simulink subsystem "DetailedBatteryModel"  (R2022b)
settings: Solver=VariableStepAuto  StartTime=0.0  StopTime=10.0  RelTol=1e-3
undefined symbols (not defined in the file): PlntBattBalSwtchThresh, PlntBattBleedRes, PlntBattCondArea, PlntBattModNumCellPar
libraries: fl_lib x584, nesl_utility_internal x386, batteryecm_lib x96, simulink x96
(part 6 of 7)

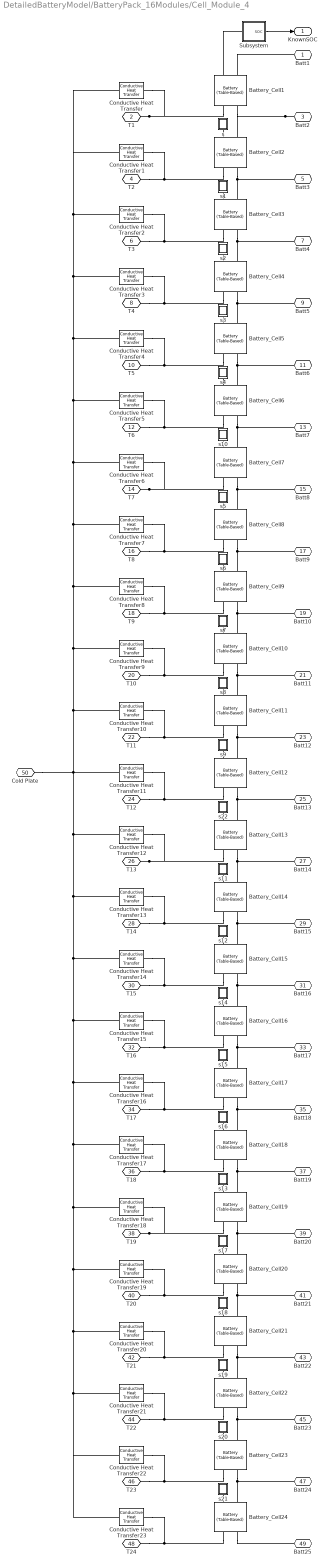
== system DetailedBatteryModel/BatteryPack_16Modules/Cell_Module_4 ==
  Battery_Cell{1..24} (24 alike) : batteryecm_lib/Battery (Table-Based)  Tag={'toolbox/physmod/battery/shared_library/m/batteryecm_lib_parts';'Battery__Table_Based_/Panasonic/NCR18650BD.xml'}  SOC_vec=[0 0.01 0.02 0.03 0.04 0.05 0.06 0.07 0.08 0.09 0.1 0.11 0.12 0.13 0.14 0.15 0.16 0.17 0.18 0.19 0.2 0.21 0.22 0.23 0.24 0.25 0.26 0.27 0.28 0.29 0.3 0.31 0.32 0.33 0.34 0.35 0.36 0.37 0.38 0.39 0.4 0.41 0.42 0.43 0.44 0.45 0.46 0.47 0.48 0.49 0.5 0.51 0.52 0.53 0.54 0.55 0.56 0.57 0.58 0.59 0.6 0.61 0.62 0.63 0.64 0.65 0.66 0.67 0.68 0.69 0.7 0.71 0.72 0.73 0.74 0.75 0.76 0.77 0.78 0.79 0.8 0.81 0.82 0.83 0.84 0.85 0.86 0.87 0.88 0.89 0.9 0.91 0.92 0.93 0.94 0.95 0.96 0.97 0.98 0.99 1]  T_dependence=simscape.enum.tablebattery.temperature_dependence.yes  prm_dir=simscape.enum.tablebattery.prm_dir.noCurrentDirectionality  T_vec=[-10 0 25 40 60] degC  V0_mat=[2.90003 2.90003 2.90003 2.90003 2.90003;2.94341 2.94341 2.94341 2.94341 2.94341;2.98679 2.98679 2.98679 2.98679 2.98679;3.04987 3.04987 3.04987 3.04987 3.04987;3.09433 3.09433 3.09433 3.09433 3.09433;3.12791 3.12791 3.12791 3.12791 3.12791;3.16031 3.16031 3.16031 3.16031 3.16031;3.20369 3.20369 3.20369 3.20369 3.20369;3.23862 3.23862 3.23862 3.23862 3.23862;3.26689 3.26689 3.26689 3.26689 3.26689;3.29115 3.29115 3.29115 3.29115 3.29115;3.31383 3.31383 3.31383 3.31383 3.31383;3.33202 3.33202 3.33202 3.33202 3.33202;3.35112 3.35112 3.35112 3.35112 3.35112;3.36833 3.36833 3.36833 3.36833 3.36833;3.38413 3.38413 3.38413 3.38413 3.38413;3.39973 3.39973 3.39973 3.39973 3.39973;3.41137 3.41137 3.41137 3.41137 3.41137;3.42149 3.42149 3.42149 3.42149 3.42149;3.43136 3.43136 3.43136 3.43136 3.43136;3.44073 3.44073 3.44073 3.44073 3.44073;3.45027 3.45027 3.45027 3.45027 3.45027;3.46068 3.46068 3.46068 3.46068 3.46068;3.47113 3.47113 3.47113 3.47113 3.47113;3.47814 3.47814 3.47814 3.47814 3.47814;3.48494 3.48494 3.48494 3.48494 3.48494;3.49199 3.49199 3.49199 3.49199 3.49199;3.49905 3.49905 3.49905 3.49905 3.49905;3.50562 3.50562 3.50562 3.50562 3.50562;3.51187 3.51187 3.51187 3.51187 3.51187;3.51861 3.51861 3.51861 3.51861 3.51861;3.52535 3.52535 3.52535 3.52535 3.52535;3.53209 3.53209 3.53209 3.53209 3.53209;3.53818 3.53818 3.53818 3.53818 3.53818;3.54353 3.54353 3.54353 3.54353 3.54353;3.54849 3.54849 3.54849 3.54849 3.54849;3.55353 3.55353 3.55353 3.55353 3.55353;3.55855 3.55855 3.55855 3.55855 3.55855;3.56357 3.56357 3.56357 3.56357 3.56357;3.56831 3.56831 3.56831 3.56831 3.56831;3.57308 3.57308 3.57308 3.57308 3.57308;3.57787 3.57787 3.57787 3.57787 3.57787;3.58264 3.58264 3.58264 3.58264 3.58264;3.58755 3.58755 3.58755 3.58755 3.58755;3.5925 3.5925 3.5925 3.5925 3.5925;3.5985 3.5985 3.5985 3.5985 3.5985;3.60496 3.60496 3.60496 3.60496 3.60496;3.61149 3.61149 3.61149 3.61149 3.61149;3.61805 3.61805 3.61805 3.61805 3.61805;3.6246 3.6246 3.6246 3.6246 3.6246;3.63116 3.63116 3.63116 3.63116 3.63116;3.63855 3.63855 3.63855 3.63855 3.63855;3.64609 3.64609 3.64609 3.64609 3.64609;3.65336 3.65336 3.65336 3.65336 3.65336;3.66064 3.66064 3.66064 3.66064 3.66064;3.66791 3.66791 3.66791 3.66791 3.66791;3.67613 3.67613 3.67613 3.67613 3.67613;3.68522 3.68522 3.68522 3.68522 3.68522;3.69443 3.69443 3.69443 3.69443 3.69443;3.70367 3.70367 3.70367 3.70367 3.70367;3.713 3.713 3.713 3.713 3.713;3.72241 3.72241 3.72241 3.72241 3.72241;3.73154 3.73154 3.73154 3.73154 3.73154;3.74037 3.74037 3.74037 3.74037 3.74037;3.7492 3.7492 3.7492 3.7492 3.7492;3.75786 3.75786 3.75786 3.75786 3.75786;3.76617 3.76617 3.76617 3.76617 3.76617;3.77556 3.77556 3.77556 3.77556 3.77556;3.78485 3.78485 3.78485 3.78485 3.78485;3.79413 3.79413 3.79413 3.79413 3.79413;3.8034 3.8034 3.8034 3.8034 3.8034;3.81149 3.81149 3.81149 3.81149 3.81149;3.81977 3.81977 3.81977 3.81977 3.81977;3.82804 3.82804 3.82804 3.82804 3.82804;3.83631 3.83631 3.83631 3.83631 3.83631;3.84472 3.84472 3.84472 3.84472 3.84472;3.85317 3.85317 3.85317 3.85317 3.85317;3.86155 3.86155 3.86155 3.86155 3.86155;3.86993 3.86993 3.86993 3.86993 3.86993;3.87831 3.87831 3.87831 3.87831 3.87831;3.88686 3.88686 3.88686 3.88686 3.88686;3.89534 3.89534 3.89534 3.89534 3.89534;3.90461 3.90461 3.90461 3.90461 3.90461;3.91454 3.91454 3.91454 3.91454 3.91454;3.92565 3.92565 3.92565 3.92565 3.92565;3.93721 3.93721 3.93721 3.93721 3.93721;3.94924 3.94924 3.94924 3.94924 3.94924;3.96155 3.96155 3.96155 3.96155 3.96155;3.97383 3.97383 3.97383 3.97383 3.97383;3.98598 3.98598 3.98598 3.98598 3.98598;3.99856 3.99856 3.99856 3.99856 3.99856;4.01117 4.01117 4.01117 4.01117 4.01117;4.02361 4.02361 4.02361 4.02361 4.02361;4.03609 4.03609 4.03609 4.03609 4.03609;4.04694 4.04694 4.04694 4.04694 4.04694;4.05695 4.05695 4.05695 4.05695 4.05695;4.06641 4.06641 4.06641 4.06641 4.06641;4.07551 4.07551 4.07551 4.07551 4.07551;4.08514 4.08514 4.08514 4.08514 4.08514;4.09447 4.09447 4.09447 4.09447 4.09447;4.10453 4.10453 4.10453 4.10453 4.10453] V  V0_vec=[2.90003 2.94341 2.98679 3.04987 3.09433 3.12791 3.16031 3.20369 3.23862 3.26689 3.29115 3.31383 3.33202 3.35112 3.36833 3.38413 3.39973 3.41137 3.42149 3.43136 3.44073 3.45027 3.46068 3.47113 3.47814 3.48494 3.49199 3.49905 3.50562 3.51187 3.51861 3.52535 3.53209 3.53818 3.54353 3.54849 3.55353 3.55855 3.56357 3.56831 3.57308 3.57787 3.58264 3.58755 3.5925 3.5985 3.60496 3.61149 3.61805 3.6246 3.63116 3.63855 3.64609 3.65336 3.66064 3.66791 3.67613 3.68522 3.69443 3.70367 3.713 3.72241 3.73154 3.74037 3.7492 3.75786 3.76617 3.77556 3.78485 3.79413 3.8034 3.81149 3.81977 3.82804 3.83631 3.84472 3.85317 3.86155 3.86993 3.87831 3.88686 3.89534 3.90461 3.91454 3.92565 3.93721 3.94924 3.96155 3.97383 3.98598 3.99856 4.01117 4.02361 4.03609 4.04694 4.05695 4.06641 4.07551 4.08514 4.09447 4.10453] V  V_range=[2.25 Inf] V  R0_mat=[0.54124 0.47218 0.1741 0.16472 0.13072;0.60048 0.51942 0.15823 0.09801 0.03241;0.57827 0.49613 0.14313 0.06257 0.00499;0.55606 0.47283 0.13285 0.0492 0.00058;0.53384 0.44953 0.12044 0.03857 0.00058;0.51163 0.42624 0.10641 0.0337 0.00058;0.48942 0.40294 0.09605 0.03258 0.00058;0.46721 0.37965 0.09162 0.03508 0.0103;0.44499 0.35635 0.08758 0.0376 0.01722;0.42278 0.33305 0.08349 0.04115 0.02235;0.40057 0.30976 0.08021 0.04338 0.0273;0.37836 0.28646 0.07738 0.04509 0.03173;0.35615 0.26317 0.07487 0.04551 0.03469;0.33393 0.24021 0.07338 0.04781 0.03783;0.31172 0.21801 0.07189 0.04948 0.04012;0.28951 0.203 0.07117 0.05069 0.04195;0.26873 0.19013 0.0704 0.05182 0.04371;0.24946 0.17834 0.06898 0.05166 0.04417;0.23189 0.16793 0.06755 0.05143 0.04397;0.21926 0.15878 0.06631 0.0513 0.04362;0.2084 0.15119 0.06509 0.05101 0.04311;0.19882 0.14534 0.06388 0.05077 0.04265;0.19282 0.14029 0.06326 0.05091 0.04272;0.18782 0.13679 0.06281 0.05124 0.04325;0.18252 0.13215 0.06182 0.05043 0.04264;0.17725 0.12766 0.06095 0.04955 0.04196;0.173 0.125 0.06025 0.04876 0.04137;0.16875 0.12234 0.05955 0.04802 0.04078;0.16459 0.11952 0.05877 0.04782 0.04033;0.16124 0.11704 0.05807 0.04752 0.03993;0.15805 0.11494 0.05761 0.04737 0.03969;0.15486 0.11285 0.05714 0.04723 0.03945;0.15212 0.11075 0.05668 0.04709 0.03921;0.15022 0.10906 0.05611 0.04673 0.03878;0.14807 0.10773 0.05546 0.04612 0.03867;0.14579 0.10628 0.0549 0.04546 0.03843;0.14353 0.10484 0.05439 0.04485 0.03821;0.14127 0.10351 0.05388 0.04423 0.03799;0.13957 0.10228 0.05337 0.04361 0.03777;0.13785 0.10097 0.0528 0.0429 0.03746;0.13614 0.09966 0.05223 0.0422 0.0367;0.13443 0.09836 0.05165 0.04151 0.03572;0.13272 0.09711 0.05106 0.04111 0.03474;0.13096 0.09591 0.05046 0.04079 0.03381;0.12918 0.09471 0.04986 0.04049 0.03288;0.12775 0.09387 0.04945 0.04053 0.03231;0.12648 0.09317 0.04913 0.04073 0.03189;0.12522 0.09249 0.04883 0.04095 0.03151;0.12398 0.09181 0.04854 0.04066 0.03136;0.12296 0.09112 0.04826 0.04006 0.03121;0.12207 0.09044 0.04797 0.03947 0.03106;0.12147 0.09003 0.04782 0.03916 0.03119;0.12091 0.08967 0.04765 0.03889 0.03136;0.12027 0.08886 0.0473 0.03854 0.03145;0.11955 0.08797 0.04695 0.03818 0.03154;0.11836 0.08708 0.04661 0.03764 0.03136;0.11749 0.08651 0.04638 0.03733 0.03126;0.1169 0.08628 0.0463 0.03731 0.03144;0.11636 0.0866 0.04625 0.03733 0.03167;0.11679 0.08693 0.04621 0.03736 0.0319;0.11639 0.08729 0.04624 0.03741 0.03216;0.11602 0.08748 0.04628 0.0375 0.03245;0.11556 0.08747 0.04628 0.03749 0.03262;0.115 0.08737 0.04623 0.03738 0.03268;0.11444 0.08726 0.04617 0.03728 0.03275;0.11413 0.08683 0.04599 0.03714 0.03276;0.11369 0.08629 0.04573 0.03712 0.03265;0.11362 0.0861 0.0457 0.03746 0.03289;0.11351 0.08597 0.04568 0.03777 0.03289;0.1134 0.08596 0.04565 0.03807 0.03285;0.11329 0.08593 0.04563 0.03837 0.0328;0.11297 0.08552 0.04535 0.03804 0.03236;0.1131 0.0855 0.0451 0.03769 0.03198;0.11323 0.08564 0.04486 0.03733 0.0316;0.11336 0.08578 0.04461 0.03698 0.03122;0.11354 0.08596 0.04446 0.03667 0.03091;0.11376 0.08614 0.04435 0.03629 0.0306;0.11421 0.08628 0.04423 0.03577 0.03027;0.11467 0.08641 0.04411 0.03525 0.02995;0.11513 0.08655 0.044 0.03473 0.02961;0.11565 0.08679 0.04372 0.03426 0.02933;0.11614 0.08704 0.04339 0.03378 0.02903;0.11689 0.08756 0.04323 0.03353 0.02899;0.11825 0.08829 0.0432 0.03328 0.02916;0.12033 0.08941 0.04344 0.03342 0.02973;0.12256 0.09067 0.04374 0.03371 0.0301;0.12495 0.09191 0.0441 0.03415 0.02981;0.12743 0.09323 0.04452 0.03468 0.0296;0.13108 0.09454 0.04494 0.03488 0.02939;0.13509 0.09581 0.0454 0.03488 0.02914;0.13924 0.09835 0.04594 0.03502 0.02907;0.14357 0.1012 0.0463 0.03517 0.02937;0.14857 0.10399 0.04649 0.03528 0.02963;0.15358 0.10679 0.04668 0.03541 0.02989;0.15894 0.10894 0.04629 0.035 0.02961;0.16451 0.11073 0.04541 0.03434 0.02892;0.17255 0.11235 0.04438 0.03375 0.02804;0.17994 0.11383 0.04326 0.03305 0.02704;0.18615 0.11422 0.04154 0.03252 0.02601;0.19123 0.11362 0.03869 0.03189 0.02484;0.17773 0.09538 0.03326 0.0315 0.0239]./PlntBattModNumCellPar Ohm  R0_vec=[0.1741 0.15823 0.14313 0.13285 0.12044 0.10641 0.09605 0.09162 0.08758 0.08349 0.08021 0.07738 0.07487 0.07338 0.07189 0.07117 0.0704 0.06898 0.06755 0.06631 0.06509 0.06388 0.06326 0.06281 0.06182 0.06095 0.06025 0.05955 0.05877 0.05807 0.05761 0.05714 0.05668 0.05611 0.05546 0.0549 0.05439 0.05388 0.05337 0.0528 0.05223 0.05165 0.05106 0.05046 0.04986 0.04945 0.04913 0.04883 0.04854 0.04826 0.04797 0.04782 0.04765 0.0473 0.04695 0.04661 0.04638 0.0463 0.04625 0.04621 0.04624 0.04628 0.04628 0.04623 0.04617 0.04599 0.04573 0.0457 0.04568 0.04565 0.04563 0.04535 0.0451 0.04486 0.04461 0.04446 0.04435 0.04423 0.04411 0.044 0.04372 0.04339 0.04323 0.0432 0.04344 0.04374 0.0441 0.04452 0.04494 0.0454 0.04594 0.0463 0.04649 0.04668 0.04629 0.04541 0.04438 0.04326 0.04154 0.03869 0.03326] Ohm  R0_dis_mat=[.0117, .0085, .009; .011, .0085, .009; .0114, .0087, .0092; .0107, .0082, .0088; .0107, .0083, .0091; .0113, .0085, .0089; .0116, .0085, .0089]./PlntBattModNumCellPar % Parameter not set Ohm  R0_dis_vec=[.0085, .0085, .0087, .0082, .0083, .0085, .0085] % Parameter not set Ohm  R0_ch_mat=[.0117, .0085, .009; .011, .0085, .009; .0114, .0087, .0092; .0107, .0082, .0088; .0107, .0083, .0091; .0113, .0085, .0089; .0116, .0085, .0089]./PlntBattModNumCellPar % Parameter not set Ohm  R0_ch_vec=[.0085, .0085, .0087, .0082, .0083, .0085, .0085] % Parameter not set Ohm  AH=3.153*PlntBattModNumCellPar hr*A  prm_leak=simscape.enum.tablebattery.prm_leak.disabled  Rleak_vec=[8000, 7000, 6000] % Parameter not set Ohm  Rleak=7e3 % Parameter not set Ohm  extrapolation_option=simscape.enum.extrapolation.nearest  SOC_port=simscape.enum.tablebattery.enable.yes  prm_dyn=simscape.enum.tablebattery.prm_dyn.off  R1_mat=[.0109, .0029, .0013; .0069, .0024, .0012; .0047, .0026, .0013; .0034, .0016, .001; .0033, .0023, .0014; .0033, .0018, .0011; .0028, .0017, .0011] % Parameter not set Ohm  R1_vec=[.0029, .0024, .0026, .0016, .0023, .0018, .0017] % Parameter not set Ohm  tau1_mat=[20, 36, 39; 31, 45, 39; 109, 105, 61; 36, 29, 26; 59, 77, 67; 40, 33, 29; 25, 39, 33] % Parameter not set s  tau1_vec=[36, 45, 105, 29, 77, 33, 39] % Parameter not set s  R2_mat=[.0109, .0029, .0013; .0069, .0024, .0012; .0047, .0026, .0013; .0034, .0016, .001; .0033, .0023, .0014; .0033, .0018, .0011; .0028, .0017, .0011] % Parameter not set Ohm  R2_vec=[.0029, .0024, .0026, .0016, .0023, .0018, .0017] % Parameter not set Ohm  tau2_mat=[20, 36, 39; 31, 45, 39; 109, 105, 61; 36, 29, 26; 59, 77, 67; 40, 33, 29; 25, 39, 33] % Parameter not set s  tau2_vec=[36, 45, 105, 29, 77, 33, 39] % Parameter not set s  R3_mat=[.0109, .0029, .0013; .0069, .0024, .0012; .0047, .0026, .0013; .0034, .0016, .001; .0033, .0023, .0014; .0033, .0018, .0011; .0028, .0017, .0011] % Parameter not set Ohm  R3_vec=[.0029, .0024, .0026, .0016, .0023, .0018, .0017] % Parameter not set Ohm  tau3_mat=[20, 36, 39; 31, 45, 39; 109, 105, 61; 36, 29, 26; 59, 77, 67; 40, 33, 29; 25, 39, 33] % Parameter not set s  tau3_vec=[36, 45, 105, 29, 77, 33, 39] % Parameter not set s  R4_mat=[.0109, .0029, .0013; .0069, .0024, .0012; .0047, .0026, .0013; .0034, .0016, .001; .0033, .0023, .0014; .0033, .0018, .0011; .0028, .0017, .0011] % Parameter not set Ohm  R4_vec=[.0029, .0024, .0026, .0016, .0023, .0018, .0017] % Parameter not set Ohm  tau4_mat=[20, 36, 39; 31, 45, 39; 109, 105, 61; 36, 29, 26; 59, 77, 67; 40, 33, 29; 25, 39, 33] % Parameter not set s  tau4_vec=[36, 45, 105, 29, 77, 33, 39] % Parameter not set s  R5_mat=[.0109, .0029, .0013; .0069, .0024, .0012; .0047, .0026, .0013; .0034, .0016, .001; .0033, .0023, .0014; .0033, .0018, .0011; .0028, .0017, .0011] % Parameter not set Ohm  R5_vec=[.0029, .0024, .0026, .0016, .0023, .0018, .0017] % Parameter not set Ohm  tau5_mat=[20, 36, 39; 31, 45, 39; 109, 105, 61; 36, 29, 26; 59, 77, 67; 40, 33, 29; 25, 39, 33] % Parameter not set s  tau5_vec=[36, 45, 105, 29, 77, 33, 39] % Parameter not set s  prm_fade=simscape.enum.tablebattery.prm_fade.disabled  N0=100 % Parameter not set  dV0=0 % Parameter not set  dR0=0 % Parameter not set  dAH=0 % Parameter not set  dRleak=0 % Parameter not set  dR1=0 % Parameter not set  dR2=0 % Parameter not set  dR3=0 % Parameter not set  dR4=0 % Parameter not set  dR5=0 % Parameter not set  N0vec=[1 5 9 13 17 21 25 29 33 37 41 45 49 53 57 61 65 69 73 77 81 85 89 93 97 101 105 109 113 117 121 125 129 133 137 141 145 149 153 157 161 165 169 173 177 181 185 189 193 197 201 205 209 213 217 221 225 229 233 237 241 245 249 253 257 261 265 269 273 277 281 285 289 293 297 301 305 309 313 317]  Tfadevec=[298.15, 323.15] % Parameter not set K  dV0vec=[0 -0.2107 -0.4072 -0.4916 -0.5781 -0.6646 -0.7487 -0.8154 -0.8801 -0.9454 -1.0127 -1.08 -1.1384 -1.1799 -1.2225 -1.2652 -1.3079 -1.3505 -1.3932 -1.4386 -1.4849 -1.5273 -1.567 -1.6067 -1.6464 -1.6889 -1.7346 -1.7803 -1.826 -1.8717 -1.9175 -1.9634 -2.0091 -2.0549 -2.1006 -2.1463 -2.1921 -2.2378 -2.2801 -2.3167 -2.3534 -2.39 -2.4267 -2.4633 -2.4999 -2.5366 -2.5732 -2.6098 -2.6449 -2.6793 -2.7137 -2.7482 -2.7826 -2.817 -2.8515 -2.8859 -2.9192 -2.9512 -2.9793 -3.0074 -3.0355 -3.0636 -3.0917 -3.1198 -3.1479 -3.1758 -3.2018 -3.2279 -3.254 -3.2801 -3.3062 -3.3323 -3.3605 -3.3912 -3.4219 -3.4526 -3.4833 -3.5141 -3.5449 -3.5756]  dR0vec=[0 0 0 0 0 0 0 0 0 0 0 0 0 0 0 0 0 0 0 0 0 0 0 0 0 0 0 0 0 0 0 0 0 0 0 0 0 0 0 0 0 0 0 0 0 0 0 0 0 0 0 0 0 0 0 0 0 0 0 0 0 0 0 0 0 0 0 0 0 0 0 0 0 0 0 0 0 0 0 0] % Parameter assumed  dAHvec=[0 -0.86 -1.713 -2.082 -2.451 -2.819 -3.188 -3.489 -3.781 -4.073 -4.365 -4.657 -4.91 -5.085 -5.26 -5.435 -5.61 -5.785 -5.96 -6.135 -6.31 -6.47 -6.62 -6.771 -6.921 -7.071 -7.221 -7.371 -7.522 -7.672 -7.822 -7.973 -8.124 -8.275 -8.426 -8.577 -8.728 -8.879 -9.018 -9.137 -9.256 -9.376 -9.495 -9.614 -9.734 -9.853 -9.972 -10.091 -10.206 -10.318 -10.431 -10.543 -10.655 -10.768 -10.88 -10.992 -11.105 -11.213 -11.308 -11.403 -11.498 -11.593 -11.687 -11.782 -11.877 -11.972 -12.059 -12.146 -12.233 -12.321 -12.408 -12.495 -12.589 -12.692 -12.794 -12.897 -12.999 -13.102 -13.205 -13.307]  dRleakvec=[0, 0, 0] % Parameter not set  dR1vec=[0, 0, 0] % Parameter not set  dR2vec=[0, 0, 0] % Parameter not set  dR3vec=[0, 0, 0] % Parameter not set  dR4vec=[0, 0, 0] % Parameter not set  dR5vec=[0, 0, 0] % Parameter not set  dV0mat=[0, 0; 0, 0; 0, 0] % Parameter not set  dR0mat=[0, 0; 0, 0; 0, 0] % Parameter not set  dAHmat=[0, 0; 0, 0; 0, 0] % Parameter not set  dRleakmat=[0, 0; 0, 0; 0, 0] % Parameter not set  dR1mat=[0, 0; 0, 0; 0, 0] % Parameter not set  dR2mat=[0, 0; 0, 0; 0, 0] % Parameter not set  dR3mat=[0, 0; 0, 0; 0, 0] % Parameter not set  dR4mat=[0, 0; 0, 0; 0, 0] % Parameter not set  dR5mat=[0, 0; 0, 0; 0, 0] % Parameter not set  prm_age_modeling=simscape.enum.tablebattery.prm_age_modeling.equation  storage_dt_age_vec=[0] % Parameter not set d  storage_T_age_vec=[273] % Parameter not set K  prm_age_OCV=simscape.enum.tablebattery.prm_age_OCV.OCV  OCV_age=0.9 % Parameter not set  SOC_age=0.6 % Parameter not set  prm_age_resistance=simscape.enum.tablebattery.prm_age.disabled  OCV_scaling_age_resistance=2.2134e6 % Parameter not set  OCV_offset_age_resistance=1.632e6 % Parameter not set  temp_exp_age_resistance=0.515833569 % Parameter not set V  t_exp_age_resistance=0.75 % Parameter not set  T_age_vec_resistance=[273.15, 298.15, 323.15] % Parameter not set K  dt_age_vec_resistance=[90, 180, 270, 360] % Parameter not set d  dR0_age_vec=[0, 0, 0] % Parameter not set  t_meas_dR0_age=100 % Parameter not set d  dR0_age_mat=[0, 0, 0; 0, 0, 0; 0, 0, 0; 0, 0, 0] % Parameter not set  prm_age_capacity=simscape.enum.tablebattery.prm_age.disabled  OCV_scaling_age_capacity=1.5097e07 % Parameter not set  OCV_offset_age_capacity=8.3625e06 % Parameter not set  temp_exp_age_capacity=0.6011 % Parameter not set V  t_exp_age_capacity=0.75 % Parameter not set  T_age_vec_capacity=[273.15, 298.15, 323.15] % Parameter not set K  dt_age_vec_capacity=[90, 180, 270, 360] % Parameter not set d  dAH_age_vec=[0, 0, 0] % Parameter not set  t_meas_dAH_age=100 % Parameter not set d  dAH_age_mat=[0, 0, 0; 0, 0, 0; 0, 0, 0; 0, 0, 0] % Parameter not set  thermal_port=simscape.enum.thermaleffects.model  temperature=298.15 % Parameter not set K  thermal_mass=44.55*PlntBattModNumCellPar % Parameter assumed J/K  i_specify=off  i_priority=None  i=0 A  i_nominal_specify=off  i_nominal_unit=A  i_nominal_value=1  v_specify=off  v_priority=None  v=0 V  v_nominal_specify=off  v_nominal_unit=V  v_nominal_value=1  stateOfCharge_specify=on  stateOfCharge_priority=High  stateOfCharge=PlntBattSocInit  stateOfCharge_nominal_specify=off  stateOfCharge_nominal_unit=1  stateOfCharge_nominal_value=1  num_cycles_specify=off  num_cycles_priority=High  num_cycles=0  num_cycles_nominal_specify=off  num_cycles_nominal_unit=1  num_cycles_nominal_value=1  cell_temperature_specify=on  cell_temperature_priority=High  cell_temperature=PlntBattTempInitDegC degC  cell_temperature_nominal_specify=off  cell_temperature_nominal_unit=K  cell_temperature_nominal_value=1
      settings: AttributesFormatString=Panasonic:NCR18650BD
  Conductive Heat Transfer{,1..23} (24 alike) : fl_lib/Thermal/Thermal Elements/Conductive Heat Transfer  thermal_type=foundation.enum.ConstantVariableTabulated.Constant  wall_geometry=foundation.enum.ConductionWallGeometry.Planar  area=PlntBattCondArea*PlntBattModNumCellPar m^2  thickness=PlntBattCondThick m  d_in=0.05 m  d_out=0.1 m  L=1 m  th_cond_min=10 W/(K*m)  th_cond=PlntBattThermCond W/(m*K)  th_cond_TLU=[413, 401, 392, 383, 371, 357, 342] W/(K*m)  temp_TLU=[200, 273, 400, 600, 800, 1000, 1200] K  T_specify=off  T_priority=None  T=0 K  T_nominal_specify=off  T_nominal_unit=K  T_nominal_value=1  Q_specify=off  Q_priority=None  Q=0 W  Q_nominal_specify=off  Q_nominal_unit=W  Q_nominal_value=1
  Subsystem : Subsystem
  s : Subsystem
  s1 : Subsystem
  s10 : Subsystem
  s11 : Subsystem
  s12 : Subsystem
  s13 : Subsystem
  s14 : Subsystem
  s15 : Subsystem
  s16 : Subsystem
  s17 : Subsystem
  s18 : Subsystem
  s19 : Subsystem
  s2 : Subsystem
  s20 : Subsystem
  s21 : Subsystem
  s22 : Subsystem
  s3 : Subsystem
  s4 : Subsystem
  s5 : Subsystem
  s6 : Subsystem
  s7 : Subsystem
  s8 : Subsystem
  s9 : Subsystem
  Batt1 : PMIOPort  Side=Right
  T1 : PMIOPort  Port=2  Side=Right
  Batt2 : PMIOPort  Port=3  Side=Right
  T2 : PMIOPort  Port=4  Side=Right
  Batt3 : PMIOPort  Port=5  Side=Right
  T3 : PMIOPort  Port=6  Side=Right
  Batt4 : PMIOPort  Port=7  Side=Right
  T4 : PMIOPort  Port=8  Side=Right
  Batt5 : PMIOPort  Port=9  Side=Right
  T5 : PMIOPort  Port=10  Side=Right
  Batt6 : PMIOPort  Port=11  Side=Right
  T6 : PMIOPort  Port=12  Side=Right
  Batt7 : PMIOPort  Port=13  Side=Right
  T7 : PMIOPort  Port=14  Side=Right
  Batt8 : PMIOPort  Port=15  Side=Right
  T8 : PMIOPort  Port=16  Side=Right
  Batt9 : PMIOPort  Port=17  Side=Right
  T9 : PMIOPort  Port=18  Side=Right
  Batt10 : PMIOPort  Port=19  Side=Right
  T10 : PMIOPort  Port=20  Side=Right
  Batt11 : PMIOPort  Port=21  Side=Right
  T11 : PMIOPort  Port=22  Side=Right
  Batt12 : PMIOPort  Port=23  Side=Right
  T12 : PMIOPort  Port=24  Side=Right
  Batt13 : PMIOPort  Port=25  Side=Right
  T13 : PMIOPort  Port=26  Side=Right
  Batt14 : PMIOPort  Port=27  Side=Right
  T14 : PMIOPort  Port=28  Side=Right
  Batt15 : PMIOPort  Port=29  Side=Right
  T15 : PMIOPort  Port=30  Side=Right
  Batt16 : PMIOPort  Port=31  Side=Right
  T16 : PMIOPort  Port=32  Side=Right
  Batt17 : PMIOPort  Port=33  Side=Right
  T17 : PMIOPort  Port=34  Side=Right
  Batt18 : PMIOPort  Port=35  Side=Right
  T18 : PMIOPort  Port=36  Side=Right
  Batt19 : PMIOPort  Port=37  Side=Right
  T19 : PMIOPort  Port=38  Side=Right
  Batt20 : PMIOPort  Port=39  Side=Right
  T20 : PMIOPort  Port=40  Side=Right
  Batt21 : PMIOPort  Port=41  Side=Right
  T21 : PMIOPort  Port=42  Side=Right
  Batt22 : PMIOPort  Port=43  Side=Right
  T22 : PMIOPort  Port=44  Side=Right
  Batt23 : PMIOPort  Port=45  Side=Right
  T23 : PMIOPort  Port=46  Side=Right
  Batt24 : PMIOPort  Port=47  Side=Right
  T24 : PMIOPort  Port=48  Side=Right
  Batt25 : PMIOPort  Port=49  Side=Right
  Cold Plate : PMIOPort  Port=50  Side=Left
  KnownSOC : Outport
  wires:
  Subsystem/1(soc) -> KnownSOC/1
  connections:
  T4/RConn1 -- Conductive Heat Transfer3/LConn1 -- Battery_Cell4/RConn2
  T2/RConn1 -- Conductive Heat Transfer1/LConn1 -- Battery_Cell2/RConn2
  T3/RConn1 -- Conductive Heat Transfer2/LConn1 -- Battery_Cell3/RConn2
  Battery_Cell6/LConn2 -- s4/LConn1
  Battery_Cell5/LConn2 -- s3/LConn1
  Battery_Cell4/LConn2 -- s2/LConn1
  Battery_Cell3/LConn2 -- s1/LConn1
  Battery_Cell2/LConn2 -- s/LConn1
  Battery_Cell1/LConn2 -- Subsystem/LConn1
  Battery_Cell2/RConn1 -- Batt3/RConn1 -- Battery_Cell3/LConn1
  Battery_Cell1/LConn1 -- Batt1/RConn1
  Battery_Cell6/RConn1 -- Batt7/RConn1 -- Battery_Cell7/LConn1
  Conductive Heat Transfer12/RConn1 -- Conductive Heat Transfer13/RConn1 -- Conductive Heat Transfer14/RConn1 -- Conductive Heat Transfer15/RConn1 -- Conductive Heat Transfer16/RConn1 -- Conductive Heat Transfer17/RConn1 -- Conductive Heat Transfer18/RConn1 -- Conductive Heat Transfer19/RConn1 -- Conductive Heat Transfer20/RConn1 -- Conductive Heat Transfer21/RConn1 -- Conductive Heat Transfer23/RConn1 -- Conductive Heat Transfer22/RConn1 -- Conductive Heat Transfer11/RConn1 -- Conductive Heat Transfer10/RConn1 -- Conductive Heat Transfer9/RConn1 -- Conductive Heat Transfer8/RConn1 -- Conductive Heat Transfer7/RConn1 -- Conductive Heat Transfer6/RConn1 -- Conductive Heat Transfer5/RConn1 -- Conductive Heat Transfer4/RConn1 -- Conductive Heat Transfer3/RConn1 -- Conductive Heat Transfer2/RConn1 -- Conductive Heat Transfer1/RConn1 -- Conductive Heat Transfer/RConn1 -- Cold Plate/RConn1
  T6/RConn1 -- Conductive Heat Transfer5/LConn1 -- Battery_Cell6/RConn2
  Batt2/RConn1 -- Battery_Cell1/RConn1 -- Battery_Cell2/LConn1
  T5/RConn1 -- Conductive Heat Transfer4/LConn1 -- Battery_Cell5/RConn2
  T1/RConn1 -- Battery_Cell1/RConn2 -- Conductive Heat Transfer/LConn1
  Battery_Cell3/RConn1 -- Batt4/RConn1 -- Battery_Cell4/LConn1
  Battery_Cell5/RConn1 -- Batt6/RConn1 -- Battery_Cell6/LConn1
  Battery_Cell4/RConn1 -- Batt5/RConn1 -- Battery_Cell5/LConn1
  T7/RConn1 -- Conductive Heat Transfer6/LConn1 -- Battery_Cell7/RConn2
  Battery_Cell7/RConn1 -- Batt8/RConn1 -- Battery_Cell8/LConn1
  T12/RConn1 -- Conductive Heat Transfer11/LConn1 -- Battery_Cell12/RConn2
  Battery_Cell11/RConn1 -- Batt12/RConn1 -- Battery_Cell12/LConn1
  Battery_Cell8/RConn1 -- Batt9/RConn1 -- Battery_Cell9/LConn1
  T10/RConn1 -- Conductive Heat Transfer9/LConn1 -- Battery_Cell10/RConn2
  Battery_Cell10/RConn1 -- Batt11/RConn1 -- Battery_Cell11/LConn1
  Battery_Cell9/RConn1 -- Batt10/RConn1 -- Battery_Cell10/LConn1
  T11/RConn1 -- Conductive Heat Transfer10/LConn1 -- Battery_Cell11/RConn2
  T8/RConn1 -- Conductive Heat Transfer7/LConn1 -- Battery_Cell8/RConn2
  T9/RConn1 -- Conductive Heat Transfer8/LConn1 -- Battery_Cell9/RConn2
  Battery_Cell11/LConn2 -- s8/LConn1
  Battery_Cell12/RConn1 -- Batt13/RConn1 -- Battery_Cell13/LConn1
  Battery_Cell10/LConn2 -- s7/LConn1
  Battery_Cell12/LConn2 -- s9/LConn1
  Battery_Cell8/LConn2 -- s5/LConn1
  Battery_Cell9/LConn2 -- s6/LConn1
  Battery_Cell7/LConn2 -- s10/LConn1
  Battery_Cell19/RConn1 -- Batt20/RConn1 -- Battery_Cell20/LConn1
  Battery_Cell13/RConn1 -- Batt14/RConn1 -- Battery_Cell14/LConn1
  T18/RConn1 -- Conductive Heat Transfer17/LConn1 -- Battery_Cell18/RConn2
  Battery_Cell20/RConn1 -- Batt21/RConn1 -- Battery_Cell21/LConn1
  T16/RConn1 -- Conductive Heat Transfer15/LConn1 -- Battery_Cell16/RConn2
  Battery_Cell15/RConn1 -- Batt16/RConn1 -- Battery_Cell16/LConn1
  Battery_Cell23/RConn1 -- Batt24/RConn1 -- Battery_Cell24/LConn1
  T14/RConn1 -- Conductive Heat Transfer13/LConn1 -- Battery_Cell14/RConn2
  T21/RConn1 -- Conductive Heat Transfer20/LConn1 -- Battery_Cell21/RConn2
  T20/RConn1 -- Conductive Heat Transfer19/LConn1 -- Battery_Cell20/RConn2
  Battery_Cell16/RConn1 -- Batt17/RConn1 -- Battery_Cell17/LConn1
  Battery_Cell22/RConn1 -- Batt23/RConn1 -- Battery_Cell23/LConn1
  Battery_Cell17/RConn1 -- Batt18/RConn1 -- Battery_Cell18/LConn1
  T22/RConn1 -- Conductive Heat Transfer21/LConn1 -- Battery_Cell22/RConn2
  T24/RConn1 -- Conductive Heat Transfer23/LConn1 -- Battery_Cell24/RConn2
  T15/RConn1 -- Conductive Heat Transfer14/LConn1 -- Battery_Cell15/RConn2
  T13/RConn1 -- Conductive Heat Transfer12/LConn1 -- Battery_Cell13/RConn2
  T17/RConn1 -- Conductive Heat Transfer16/LConn1 -- Battery_Cell17/RConn2
  Battery_Cell21/RConn1 -- Batt22/RConn1 -- Battery_Cell22/LConn1
  Battery_Cell18/RConn1 -- Batt19/RConn1 -- Battery_Cell19/LConn1
  T19/RConn1 -- Conductive Heat Transfer18/LConn1 -- Battery_Cell19/RConn2
  T23/RConn1 -- Conductive Heat Transfer22/LConn1 -- Battery_Cell23/RConn2
  Battery_Cell14/RConn1 -- Batt15/RConn1 -- Battery_Cell15/LConn1
  Battery_Cell22/LConn2 -- s19/LConn1
  Battery_Cell17/LConn2 -- s15/LConn1
  Battery_Cell16/LConn2 -- s14/LConn1
  Battery_Cell24/LConn2 -- s21/LConn1
  Battery_Cell20/LConn2 -- s17/LConn1
  Battery_Cell18/LConn2 -- s16/LConn1
  Battery_Cell23/LConn2 -- s20/LConn1
  Battery_Cell14/LConn2 -- s11/LConn1
  Battery_Cell19/LConn2 -- s13/LConn1
  Battery_Cell15/LConn2 -- s12/LConn1
  Battery_Cell24/RConn1 -- Batt25/RConn1
  Battery_Cell21/LConn2 -- s18/LConn1
  Battery_Cell13/LConn2 -- s22/LConn1

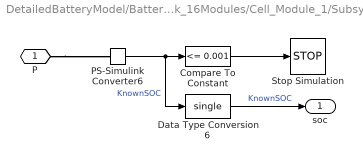
== system DetailedBatteryModel/BatteryPack_16Modules/Cell_Module_1/Subsystem ==
  Compare To Constant : simulink/Logic and Bit Operations/Compare To Constant  relop=<=  const=0.001  OutDataTypeStr=boolean
  Data Type Conversion6 : DataTypeConversion  OutDataTypeStr=single  SaturateOnIntegerOverflow=off  RndMeth=Floor
  PS-Simulink Converter6 : nesl_utility_internal/PS-Simulink Converter  PhysicalDomain=network_engine_domain  SubClassName=ps_output  LeftPortType=input  RightPortType=output  PseudoPeriodic=off  Frequencies=[]  VectorFormat=1-D array  Unit=1  AffineConversion=off
  Stop Simulation : Stop
  P : PMIOPort  Side=Left
  soc : Outport
  wires:
  Data Type Conversion6/1 -> soc/1  "KnownSOC"
  PS-Simulink Converter6/1 -> Compare To Constant/1, Data Type Conversion6/1  "KnownSOC"
  Compare To Constant/1 -> Stop Simulation/1
  connections:
  P/RConn1 -- PS-Simulink Converter6/LConn1

== system DetailedBatteryModel/BatteryPack_16Modules/Cell_Module_1/s ==
  Compare To Constant1 : simulink/Logic and Bit Operations/Compare To Constant  relop=<=  const=0.001  OutDataTypeStr=boolean
  PS-Simulink Converter7 : nesl_utility_internal/PS-Simulink Converter  PhysicalDomain=network_engine_domain  SubClassName=ps_output  LeftPortType=input  RightPortType=output  PseudoPeriodic=off  Frequencies=[]  VectorFormat=1-D array  Unit=1  AffineConversion=off
  Stop Simulation1 : Stop
  p : PMIOPort  Side=Left
  wires:
  PS-Simulink Converter7/1 -> Compare To Constant1/1
  Compare To Constant1/1 -> Stop Simulation1/1
  connections:
  PS-Simulink Converter7/LConn1 -- p/RConn1

== system DetailedBatteryModel/BatteryPack_16Modules/Cell_Module_1/s1 ==
  Compare To Constant2 : simulink/Logic and Bit Operations/Compare To Constant  relop=<=  const=0.001  OutDataTypeStr=boolean
  PS-Simulink Converter8 : nesl_utility_internal/PS-Simulink Converter  PhysicalDomain=network_engine_domain  SubClassName=ps_output  LeftPortType=input  RightPortType=output  PseudoPeriodic=off  Frequencies=[]  VectorFormat=1-D array  Unit=1  AffineConversion=off
  Stop Simulation2 : Stop
  p : PMIOPort  Side=Left
  wires:
  Compare To Constant2/1 -> Stop Simulation2/1
  PS-Simulink Converter8/1 -> Compare To Constant2/1
  connections:
  PS-Simulink Converter8/LConn1 -- p/RConn1

== system DetailedBatteryModel/BatteryPack_16Modules/Cell_Module_1/s10 ==
  Compare To Constant5 : simulink/Logic and Bit Operations/Compare To Constant  relop=<=  const=0.001  OutDataTypeStr=boolean
  PS-Simulink Converter11 : nesl_utility_internal/PS-Simulink Converter  PhysicalDomain=network_engine_domain  SubClassName=ps_output  LeftPortType=input  RightPortType=output  PseudoPeriodic=off  Frequencies=[]  VectorFormat=1-D array  Unit=1  AffineConversion=off
  Stop Simulation5 : Stop
  p : PMIOPort  Side=Left
  wires:
  Compare To Constant5/1 -> Stop Simulation5/1
  PS-Simulink Converter11/1 -> Compare To Constant5/1
  connections:
  PS-Simulink Converter11/LConn1 -- p/RConn1

== system DetailedBatteryModel/BatteryPack_16Modules/Cell_Module_1/s11 ==
  Compare To Constant1 : simulink/Logic and Bit Operations/Compare To Constant  relop=<=  const=0.001  OutDataTypeStr=boolean
  PS-Simulink Converter7 : nesl_utility_internal/PS-Simulink Converter  PhysicalDomain=network_engine_domain  SubClassName=ps_output  LeftPortType=input  RightPortType=output  PseudoPeriodic=off  Frequencies=[]  VectorFormat=1-D array  Unit=1  AffineConversion=off
  Stop Simulation1 : Stop
  p : PMIOPort  Side=Left
  wires:
  PS-Simulink Converter7/1 -> Compare To Constant1/1
  Compare To Constant1/1 -> Stop Simulation1/1
  connections:
  PS-Simulink Converter7/LConn1 -- p/RConn1

== system DetailedBatteryModel/BatteryPack_16Modules/Cell_Module_1/s12 ==
  Compare To Constant2 : simulink/Logic and Bit Operations/Compare To Constant  relop=<=  const=0.001  OutDataTypeStr=boolean
  PS-Simulink Converter8 : nesl_utility_internal/PS-Simulink Converter  PhysicalDomain=network_engine_domain  SubClassName=ps_output  LeftPortType=input  RightPortType=output  PseudoPeriodic=off  Frequencies=[]  VectorFormat=1-D array  Unit=1  AffineConversion=off
  Stop Simulation2 : Stop
  p : PMIOPort  Side=Left
  wires:
  Compare To Constant2/1 -> Stop Simulation2/1
  PS-Simulink Converter8/1 -> Compare To Constant2/1
  connections:
  PS-Simulink Converter8/LConn1 -- p/RConn1

== system DetailedBatteryModel/BatteryPack_16Modules/Cell_Module_1/s13 ==
  Compare To Constant5 : simulink/Logic and Bit Operations/Compare To Constant  relop=<=  const=0.001  OutDataTypeStr=boolean
  PS-Simulink Converter11 : nesl_utility_internal/PS-Simulink Converter  PhysicalDomain=network_engine_domain  SubClassName=ps_output  LeftPortType=input  RightPortType=output  PseudoPeriodic=off  Frequencies=[]  VectorFormat=1-D array  Unit=1  AffineConversion=off
  Stop Simulation5 : Stop
  p : PMIOPort  Side=Left
  wires:
  Compare To Constant5/1 -> Stop Simulation5/1
  PS-Simulink Converter11/1 -> Compare To Constant5/1
  connections:
  PS-Simulink Converter11/LConn1 -- p/RConn1

== system DetailedBatteryModel/BatteryPack_16Modules/Cell_Module_1/s14 ==
  Compare To Constant3 : simulink/Logic and Bit Operations/Compare To Constant  relop=<=  const=0.001  OutDataTypeStr=boolean
  PS-Simulink Converter9 : nesl_utility_internal/PS-Simulink Converter  PhysicalDomain=network_engine_domain  SubClassName=ps_output  LeftPortType=input  RightPortType=output  PseudoPeriodic=off  Frequencies=[]  VectorFormat=1-D array  Unit=1  AffineConversion=off
  Stop Simulation3 : Stop
  p : PMIOPort  Side=Left
  wires:
  PS-Simulink Converter9/1 -> Compare To Constant3/1
  Compare To Constant3/1 -> Stop Simulation3/1
  connections:
  PS-Simulink Converter9/LConn1 -- p/RConn1

== system DetailedBatteryModel/BatteryPack_16Modules/Cell_Module_1/s15 ==
  Compare To Constant4 : simulink/Logic and Bit Operations/Compare To Constant  relop=<=  const=0.001  OutDataTypeStr=boolean
  PS-Simulink Converter10 : nesl_utility_internal/PS-Simulink Converter  PhysicalDomain=network_engine_domain  SubClassName=ps_output  LeftPortType=input  RightPortType=output  PseudoPeriodic=off  Frequencies=[]  VectorFormat=1-D array  Unit=1  AffineConversion=off
  Stop Simulation4 : Stop
  p : PMIOPort  Side=Left
  wires:
  PS-Simulink Converter10/1 -> Compare To Constant4/1
  Compare To Constant4/1 -> Stop Simulation4/1
  connections:
  PS-Simulink Converter10/LConn1 -- p/RConn1

== system DetailedBatteryModel/BatteryPack_16Modules/Cell_Module_1/s16 ==
  Compare To Constant5 : simulink/Logic and Bit Operations/Compare To Constant  relop=<=  const=0.001  OutDataTypeStr=boolean
  PS-Simulink Converter11 : nesl_utility_internal/PS-Simulink Converter  PhysicalDomain=network_engine_domain  SubClassName=ps_output  LeftPortType=input  RightPortType=output  PseudoPeriodic=off  Frequencies=[]  VectorFormat=1-D array  Unit=1  AffineConversion=off
  Stop Simulation5 : Stop
  p : PMIOPort  Side=Left
  wires:
  PS-Simulink Converter11/1 -> Compare To Constant5/1
  Compare To Constant5/1 -> Stop Simulation5/1
  connections:
  PS-Simulink Converter11/LConn1 -- p/RConn1

== system DetailedBatteryModel/BatteryPack_16Modules/Cell_Module_1/s17 ==
  Compare To Constant1 : simulink/Logic and Bit Operations/Compare To Constant  relop=<=  const=0.001  OutDataTypeStr=boolean
  PS-Simulink Converter7 : nesl_utility_internal/PS-Simulink Converter  PhysicalDomain=network_engine_domain  SubClassName=ps_output  LeftPortType=input  RightPortType=output  PseudoPeriodic=off  Frequencies=[]  VectorFormat=1-D array  Unit=1  AffineConversion=off
  Stop Simulation1 : Stop
  p : PMIOPort  Side=Left
  wires:
  PS-Simulink Converter7/1 -> Compare To Constant1/1
  Compare To Constant1/1 -> Stop Simulation1/1
  connections:
  PS-Simulink Converter7/LConn1 -- p/RConn1

== system DetailedBatteryModel/BatteryPack_16Modules/Cell_Module_1/s18 ==
  Compare To Constant2 : simulink/Logic and Bit Operations/Compare To Constant  relop=<=  const=0.001  OutDataTypeStr=boolean
  PS-Simulink Converter8 : nesl_utility_internal/PS-Simulink Converter  PhysicalDomain=network_engine_domain  SubClassName=ps_output  LeftPortType=input  RightPortType=output  PseudoPeriodic=off  Frequencies=[]  VectorFormat=1-D array  Unit=1  AffineConversion=off
  Stop Simulation2 : Stop
  p : PMIOPort  Side=Left
  wires:
  Compare To Constant2/1 -> Stop Simulation2/1
  PS-Simulink Converter8/1 -> Compare To Constant2/1
  connections:
  PS-Simulink Converter8/LConn1 -- p/RConn1

== system DetailedBatteryModel/BatteryPack_16Modules/Cell_Module_1/s19 ==
  Compare To Constant3 : simulink/Logic and Bit Operations/Compare To Constant  relop=<=  const=0.001  OutDataTypeStr=boolean
  PS-Simulink Converter9 : nesl_utility_internal/PS-Simulink Converter  PhysicalDomain=network_engine_domain  SubClassName=ps_output  LeftPortType=input  RightPortType=output  PseudoPeriodic=off  Frequencies=[]  VectorFormat=1-D array  Unit=1  AffineConversion=off
  Stop Simulation3 : Stop
  p : PMIOPort  Side=Left
  wires:
  PS-Simulink Converter9/1 -> Compare To Constant3/1
  Compare To Constant3/1 -> Stop Simulation3/1
  connections:
  PS-Simulink Converter9/LConn1 -- p/RConn1

== system DetailedBatteryModel/BatteryPack_16Modules/Cell_Module_1/s2 ==
  Compare To Constant3 : simulink/Logic and Bit Operations/Compare To Constant  relop=<=  const=0.001  OutDataTypeStr=boolean
  PS-Simulink Converter9 : nesl_utility_internal/PS-Simulink Converter  PhysicalDomain=network_engine_domain  SubClassName=ps_output  LeftPortType=input  RightPortType=output  PseudoPeriodic=off  Frequencies=[]  VectorFormat=1-D array  Unit=1  AffineConversion=off
  Stop Simulation3 : Stop
  p : PMIOPort  Side=Left
  wires:
  PS-Simulink Converter9/1 -> Compare To Constant3/1
  Compare To Constant3/1 -> Stop Simulation3/1
  connections:
  PS-Simulink Converter9/LConn1 -- p/RConn1

== system DetailedBatteryModel/BatteryPack_16Modules/Cell_Module_1/s20 ==
  Compare To Constant4 : simulink/Logic and Bit Operations/Compare To Constant  relop=<=  const=0.001  OutDataTypeStr=boolean
  PS-Simulink Converter10 : nesl_utility_internal/PS-Simulink Converter  PhysicalDomain=network_engine_domain  SubClassName=ps_output  LeftPortType=input  RightPortType=output  PseudoPeriodic=off  Frequencies=[]  VectorFormat=1-D array  Unit=1  AffineConversion=off
  Stop Simulation4 : Stop
  p : PMIOPort  Side=Left
  wires:
  PS-Simulink Converter10/1 -> Compare To Constant4/1
  Compare To Constant4/1 -> Stop Simulation4/1
  connections:
  PS-Simulink Converter10/LConn1 -- p/RConn1

== system DetailedBatteryModel/BatteryPack_16Modules/Cell_Module_1/s21 ==
  Compare To Constant5 : simulink/Logic and Bit Operations/Compare To Constant  relop=<=  const=0.001  OutDataTypeStr=boolean
  PS-Simulink Converter11 : nesl_utility_internal/PS-Simulink Converter  PhysicalDomain=network_engine_domain  SubClassName=ps_output  LeftPortType=input  RightPortType=output  PseudoPeriodic=off  Frequencies=[]  VectorFormat=1-D array  Unit=1  AffineConversion=off
  Stop Simulation5 : Stop
  p : PMIOPort  Side=Left
  wires:
  PS-Simulink Converter11/1 -> Compare To Constant5/1
  Compare To Constant5/1 -> Stop Simulation5/1
  connections:
  PS-Simulink Converter11/LConn1 -- p/RConn1

== system DetailedBatteryModel/BatteryPack_16Modules/Cell_Module_1/s22 ==
  Compare To Constant5 : simulink/Logic and Bit Operations/Compare To Constant  relop=<=  const=0.001  OutDataTypeStr=boolean
  PS-Simulink Converter11 : nesl_utility_internal/PS-Simulink Converter  PhysicalDomain=network_engine_domain  SubClassName=ps_output  LeftPortType=input  RightPortType=output  PseudoPeriodic=off  Frequencies=[]  VectorFormat=1-D array  Unit=1  AffineConversion=off
  Stop Simulation5 : Stop
  p : PMIOPort  Side=Left
  wires:
  Compare To Constant5/1 -> Stop Simulation5/1
  PS-Simulink Converter11/1 -> Compare To Constant5/1
  connections:
  PS-Simulink Converter11/LConn1 -- p/RConn1

== system DetailedBatteryModel/BatteryPack_16Modules/Cell_Module_1/s3 ==
  Compare To Constant4 : simulink/Logic and Bit Operations/Compare To Constant  relop=<=  const=0.001  OutDataTypeStr=boolean
  PS-Simulink Converter10 : nesl_utility_internal/PS-Simulink Converter  PhysicalDomain=network_engine_domain  SubClassName=ps_output  LeftPortType=input  RightPortType=output  PseudoPeriodic=off  Frequencies=[]  VectorFormat=1-D array  Unit=1  AffineConversion=off
  Stop Simulation4 : Stop
  p : PMIOPort  Side=Left
  wires:
  PS-Simulink Converter10/1 -> Compare To Constant4/1
  Compare To Constant4/1 -> Stop Simulation4/1
  connections:
  PS-Simulink Converter10/LConn1 -- p/RConn1

== system DetailedBatteryModel/BatteryPack_16Modules/Cell_Module_1/s4 ==
  Compare To Constant5 : simulink/Logic and Bit Operations/Compare To Constant  relop=<=  const=0.001  OutDataTypeStr=boolean
  PS-Simulink Converter11 : nesl_utility_internal/PS-Simulink Converter  PhysicalDomain=network_engine_domain  SubClassName=ps_output  LeftPortType=input  RightPortType=output  PseudoPeriodic=off  Frequencies=[]  VectorFormat=1-D array  Unit=1  AffineConversion=off
  Stop Simulation5 : Stop
  p : PMIOPort  Side=Left
  wires:
  PS-Simulink Converter11/1 -> Compare To Constant5/1
  Compare To Constant5/1 -> Stop Simulation5/1
  connections:
  PS-Simulink Converter11/LConn1 -- p/RConn1

== system DetailedBatteryModel/BatteryPack_16Modules/Cell_Module_1/s5 ==
  Compare To Constant1 : simulink/Logic and Bit Operations/Compare To Constant  relop=<=  const=0.001  OutDataTypeStr=boolean
  PS-Simulink Converter7 : nesl_utility_internal/PS-Simulink Converter  PhysicalDomain=network_engine_domain  SubClassName=ps_output  LeftPortType=input  RightPortType=output  PseudoPeriodic=off  Frequencies=[]  VectorFormat=1-D array  Unit=1  AffineConversion=off
  Stop Simulation1 : Stop
  p : PMIOPort  Side=Left
  wires:
  PS-Simulink Converter7/1 -> Compare To Constant1/1
  Compare To Constant1/1 -> Stop Simulation1/1
  connections:
  PS-Simulink Converter7/LConn1 -- p/RConn1

== system DetailedBatteryModel/BatteryPack_16Modules/Cell_Module_1/s6 ==
  Compare To Constant2 : simulink/Logic and Bit Operations/Compare To Constant  relop=<=  const=0.001  OutDataTypeStr=boolean
  PS-Simulink Converter8 : nesl_utility_internal/PS-Simulink Converter  PhysicalDomain=network_engine_domain  SubClassName=ps_output  LeftPortType=input  RightPortType=output  PseudoPeriodic=off  Frequencies=[]  VectorFormat=1-D array  Unit=1  AffineConversion=off
  Stop Simulation2 : Stop
  p : PMIOPort  Side=Left
  wires:
  Compare To Constant2/1 -> Stop Simulation2/1
  PS-Simulink Converter8/1 -> Compare To Constant2/1
  connections:
  PS-Simulink Converter8/LConn1 -- p/RConn1

== system DetailedBatteryModel/BatteryPack_16Modules/Cell_Module_1/s7 ==
  Compare To Constant3 : simulink/Logic and Bit Operations/Compare To Constant  relop=<=  const=0.001  OutDataTypeStr=boolean
  PS-Simulink Converter9 : nesl_utility_internal/PS-Simulink Converter  PhysicalDomain=network_engine_domain  SubClassName=ps_output  LeftPortType=input  RightPortType=output  PseudoPeriodic=off  Frequencies=[]  VectorFormat=1-D array  Unit=1  AffineConversion=off
  Stop Simulation3 : Stop
  p : PMIOPort  Side=Left
  wires:
  PS-Simulink Converter9/1 -> Compare To Constant3/1
  Compare To Constant3/1 -> Stop Simulation3/1
  connections:
  PS-Simulink Converter9/LConn1 -- p/RConn1

== system DetailedBatteryModel/BatteryPack_16Modules/Cell_Module_1/s8 ==
  Compare To Constant4 : simulink/Logic and Bit Operations/Compare To Constant  relop=<=  const=0.001  OutDataTypeStr=boolean
  PS-Simulink Converter10 : nesl_utility_internal/PS-Simulink Converter  PhysicalDomain=network_engine_domain  SubClassName=ps_output  LeftPortType=input  RightPortType=output  PseudoPeriodic=off  Frequencies=[]  VectorFormat=1-D array  Unit=1  AffineConversion=off
  Stop Simulation4 : Stop
  p : PMIOPort  Side=Left
  wires:
  PS-Simulink Converter10/1 -> Compare To Constant4/1
  Compare To Constant4/1 -> Stop Simulation4/1
  connections:
  PS-Simulink Converter10/LConn1 -- p/RConn1

== system DetailedBatteryModel/BatteryPack_16Modules/Cell_Module_1/s9 ==
  Compare To Constant5 : simulink/Logic and Bit Operations/Compare To Constant  relop=<=  const=0.001  OutDataTypeStr=boolean
  PS-Simulink Converter11 : nesl_utility_internal/PS-Simulink Converter  PhysicalDomain=network_engine_domain  SubClassName=ps_output  LeftPortType=input  RightPortType=output  PseudoPeriodic=off  Frequencies=[]  VectorFormat=1-D array  Unit=1  AffineConversion=off
  Stop Simulation5 : Stop
  p : PMIOPort  Side=Left
  wires:
  PS-Simulink Converter11/1 -> Compare To Constant5/1
  Compare To Constant5/1 -> Stop Simulation5/1
  connections:
  PS-Simulink Converter11/LConn1 -- p/RConn1

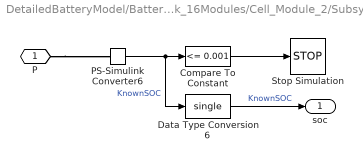
== system DetailedBatteryModel/BatteryPack_16Modules/Cell_Module_2/Subsystem ==
  Compare To Constant : simulink/Logic and Bit Operations/Compare To Constant  relop=<=  const=0.001  OutDataTypeStr=boolean
  Data Type Conversion6 : DataTypeConversion  OutDataTypeStr=single  SaturateOnIntegerOverflow=off  RndMeth=Floor
  PS-Simulink Converter6 : nesl_utility_internal/PS-Simulink Converter  PhysicalDomain=network_engine_domain  SubClassName=ps_output  LeftPortType=input  RightPortType=output  PseudoPeriodic=off  Frequencies=[]  VectorFormat=1-D array  Unit=1  AffineConversion=off
  Stop Simulation : Stop
  P : PMIOPort  Side=Left
  soc : Outport
  wires:
  Data Type Conversion6/1 -> soc/1  "KnownSOC"
  PS-Simulink Converter6/1 -> Compare To Constant/1, Data Type Conversion6/1  "KnownSOC"
  Compare To Constant/1 -> Stop Simulation/1
  connections:
  P/RConn1 -- PS-Simulink Converter6/LConn1

== system DetailedBatteryModel/BatteryPack_16Modules/Cell_Module_2/s ==
  Compare To Constant1 : simulink/Logic and Bit Operations/Compare To Constant  relop=<=  const=0.001  OutDataTypeStr=boolean
  PS-Simulink Converter7 : nesl_utility_internal/PS-Simulink Converter  PhysicalDomain=network_engine_domain  SubClassName=ps_output  LeftPortType=input  RightPortType=output  PseudoPeriodic=off  Frequencies=[]  VectorFormat=1-D array  Unit=1  AffineConversion=off
  Stop Simulation1 : Stop
  p : PMIOPort  Side=Left
  wires:
  PS-Simulink Converter7/1 -> Compare To Constant1/1
  Compare To Constant1/1 -> Stop Simulation1/1
  connections:
  PS-Simulink Converter7/LConn1 -- p/RConn1

== system DetailedBatteryModel/BatteryPack_16Modules/Cell_Module_2/s1 ==
  Compare To Constant2 : simulink/Logic and Bit Operations/Compare To Constant  relop=<=  const=0.001  OutDataTypeStr=boolean
  PS-Simulink Converter8 : nesl_utility_internal/PS-Simulink Converter  PhysicalDomain=network_engine_domain  SubClassName=ps_output  LeftPortType=input  RightPortType=output  PseudoPeriodic=off  Frequencies=[]  VectorFormat=1-D array  Unit=1  AffineConversion=off
  Stop Simulation2 : Stop
  p : PMIOPort  Side=Left
  wires:
  Compare To Constant2/1 -> Stop Simulation2/1
  PS-Simulink Converter8/1 -> Compare To Constant2/1
  connections:
  PS-Simulink Converter8/LConn1 -- p/RConn1

== system DetailedBatteryModel/BatteryPack_16Modules/Cell_Module_2/s10 ==
  Compare To Constant5 : simulink/Logic and Bit Operations/Compare To Constant  relop=<=  const=0.001  OutDataTypeStr=boolean
  PS-Simulink Converter11 : nesl_utility_internal/PS-Simulink Converter  PhysicalDomain=network_engine_domain  SubClassName=ps_output  LeftPortType=input  RightPortType=output  PseudoPeriodic=off  Frequencies=[]  VectorFormat=1-D array  Unit=1  AffineConversion=off
  Stop Simulation5 : Stop
  p : PMIOPort  Side=Left
  wires:
  Compare To Constant5/1 -> Stop Simulation5/1
  PS-Simulink Converter11/1 -> Compare To Constant5/1
  connections:
  PS-Simulink Converter11/LConn1 -- p/RConn1

== system DetailedBatteryModel/BatteryPack_16Modules/Cell_Module_2/s11 ==
  Compare To Constant1 : simulink/Logic and Bit Operations/Compare To Constant  relop=<=  const=0.001  OutDataTypeStr=boolean
  PS-Simulink Converter7 : nesl_utility_internal/PS-Simulink Converter  PhysicalDomain=network_engine_domain  SubClassName=ps_output  LeftPortType=input  RightPortType=output  PseudoPeriodic=off  Frequencies=[]  VectorFormat=1-D array  Unit=1  AffineConversion=off
  Stop Simulation1 : Stop
  p : PMIOPort  Side=Left
  wires:
  PS-Simulink Converter7/1 -> Compare To Constant1/1
  Compare To Constant1/1 -> Stop Simulation1/1
  connections:
  PS-Simulink Converter7/LConn1 -- p/RConn1

== system DetailedBatteryModel/BatteryPack_16Modules/Cell_Module_2/s12 ==
  Compare To Constant2 : simulink/Logic and Bit Operations/Compare To Constant  relop=<=  const=0.001  OutDataTypeStr=boolean
  PS-Simulink Converter8 : nesl_utility_internal/PS-Simulink Converter  PhysicalDomain=network_engine_domain  SubClassName=ps_output  LeftPortType=input  RightPortType=output  PseudoPeriodic=off  Frequencies=[]  VectorFormat=1-D array  Unit=1  AffineConversion=off
  Stop Simulation2 : Stop
  p : PMIOPort  Side=Left
  wires:
  Compare To Constant2/1 -> Stop Simulation2/1
  PS-Simulink Converter8/1 -> Compare To Constant2/1
  connections:
  PS-Simulink Converter8/LConn1 -- p/RConn1

== system DetailedBatteryModel/BatteryPack_16Modules/Cell_Module_2/s13 ==
  Compare To Constant5 : simulink/Logic and Bit Operations/Compare To Constant  relop=<=  const=0.001  OutDataTypeStr=boolean
  PS-Simulink Converter11 : nesl_utility_internal/PS-Simulink Converter  PhysicalDomain=network_engine_domain  SubClassName=ps_output  LeftPortType=input  RightPortType=output  PseudoPeriodic=off  Frequencies=[]  VectorFormat=1-D array  Unit=1  AffineConversion=off
  Stop Simulation5 : Stop
  p : PMIOPort  Side=Left
  wires:
  Compare To Constant5/1 -> Stop Simulation5/1
  PS-Simulink Converter11/1 -> Compare To Constant5/1
  connections:
  PS-Simulink Converter11/LConn1 -- p/RConn1

== system DetailedBatteryModel/BatteryPack_16Modules/Cell_Module_2/s14 ==
  Compare To Constant3 : simulink/Logic and Bit Operations/Compare To Constant  relop=<=  const=0.001  OutDataTypeStr=boolean
  PS-Simulink Converter9 : nesl_utility_internal/PS-Simulink Converter  PhysicalDomain=network_engine_domain  SubClassName=ps_output  LeftPortType=input  RightPortType=output  PseudoPeriodic=off  Frequencies=[]  VectorFormat=1-D array  Unit=1  AffineConversion=off
  Stop Simulation3 : Stop
  p : PMIOPort  Side=Left
  wires:
  PS-Simulink Converter9/1 -> Compare To Constant3/1
  Compare To Constant3/1 -> Stop Simulation3/1
  connections:
  PS-Simulink Converter9/LConn1 -- p/RConn1
